simulink model "blockdemo"  (Simulink 6.3)
settings: Solver=ode45  StartTime=0.0  StopTime=100  RelTol=1e-3
InitFcn:
  | %% DSPBuilder Start
  | alt_dspbuilder_update_model(bdroot)
  | %% DSPBuilder End
libraries: allblocks_alteradspbuilder2 x5
settings Model: Creator=cpurcell  LastModifiedBy=delphick
settings DebuggingCC: MultiTaskDSMMsg=error

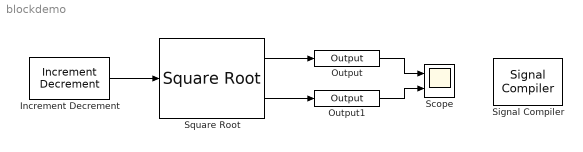
== system blockdemo ==
  Increment Decrement : allblocks_alteradspbuilder2/Increment Decrement  BusType=Unsigned Integer  bwl=6  bwr=8  SpecifyClock=off  clr_value=0  direction=Increment  phase_selection=1  use_ena=off  use_sclr=off
  Output : allblocks_alteradspbuilder2/Output  iofile=C:\workspace_clean\Documentation\DesignExamples\Tutorials\UnitBlocks\Arithmetic\SquareRoot\tb_blockdemo\blockdemo_Output.capture  BusType=Inferred  bwl=8  bwr=0  PORTTYPE=Output
  Output1 : allblocks_alteradspbuilder2/Output  iofile=C:\workspace_clean\Documentation\DesignExamples\Tutorials\UnitBlocks\Arithmetic\SquareRoot\tb_blockdemo\blockdemo_Output1.capture  BusType=Inferred  bwl=8  bwr=0  PORTTYPE=Output
  Scope : Scope  NumInputPorts=2
      settings: TimeRange=100  YMin=0~0  YMax=8~15
  Signal Compiler : allblocks_alteradspbuilder2/Signal Compiler  DeviceFamily=Stratix IV  DeviceName=AUTO  EnableSignalTap=off  SignalTapDepth=128  UseBoardBlock=off  StpUseDefaultClock=on  StpClock=clock
  Square Root : allblocks_alteradspbuilder2/Square Root  BusType=Unsigned Integer  bwl=6  bwr=0  pipeline=1  use_remain=on  use_ena=off  use_aclr=off
  wires:
  Increment Decrement/1 -> Square Root/1
  Square Root/1 -> Output/1
  Square Root/2 -> Output1/1
  Output/1 -> Scope/1
  Output1/1 -> Scope/2
